simulink model "modelo"  (R2017b)
settings: Solver=VariableStepAuto  StartTime=0.0  StopTime=20  RelTol=1e-3
settings Model: Creator=javi  LastModifiedBy=javi

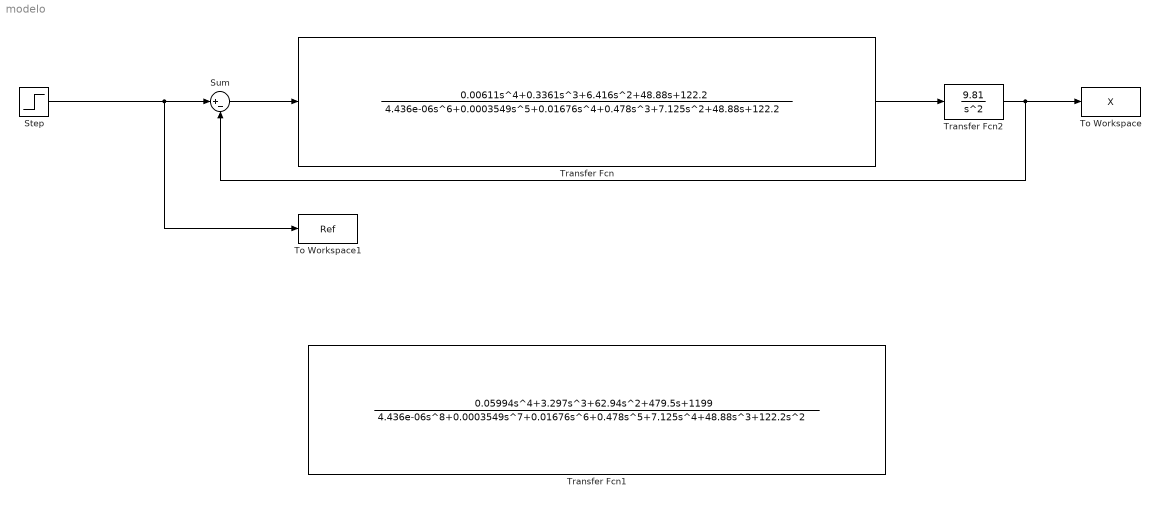
== system modelo ==
  Step : Step  Time=10  SampleTime=0
  Sum : Sum  Inputs=|+-
  To Workspace : ToWorkspace  VariableName=X  SampleTime=-1
  To Workspace1 : ToWorkspace  VariableName=Ref  SampleTime=-1
  Transfer Fcn : TransferFcn  Numerator=[0.00611 0.3361 6.416 48.88 122.2]  Denominator=[4.436e-06 0.0003549 0.01676 0.478 7.125 48.88 122.2]
  Transfer Fcn1 : TransferFcn  Numerator=[0.05994 3.297 62.94 479.5 1199]  Denominator=[4.436e-06 0.0003549 0.01676 0.478 7.125 48.88 122.2 0 0]
  Transfer Fcn2 : TransferFcn  Numerator=[9.81]  Denominator=[1 0 0]
  wires:
  Step/1 -> Sum/1, To Workspace1/1
  Transfer Fcn/1 -> Transfer Fcn2/1
  Transfer Fcn2/1 -> Sum/2, To Workspace/1
  Sum/1 -> Transfer Fcn/1
